simulink model "ImpedanceControl"  (R2020b)
settings: Solver=VariableStepAuto  StartTime=0.0  StopTime=10.0  RelTol=1e-3
libraries: simulink x1
settings Model: Creator=vac  LastModifiedBy=vac

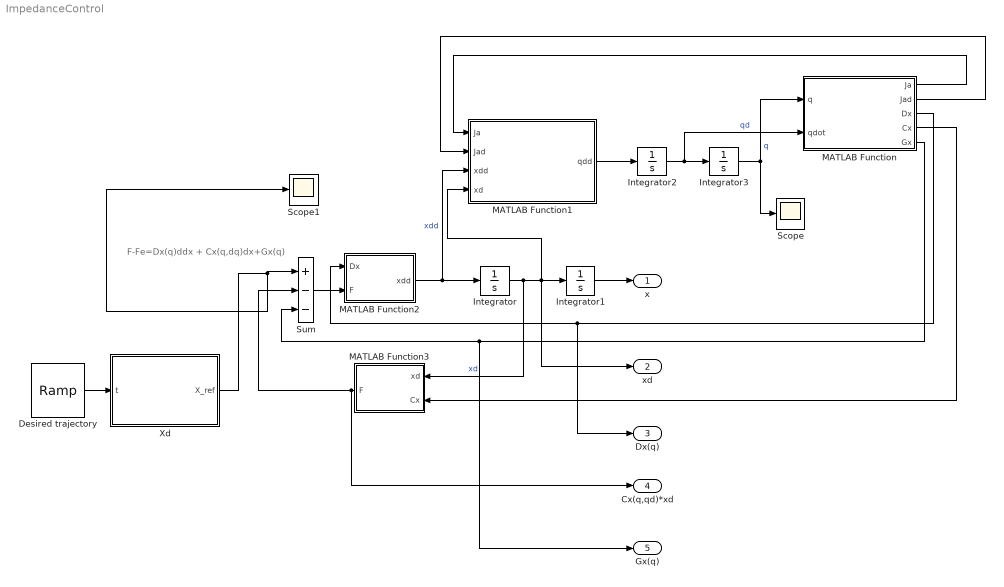
== system ImpedanceControl ==
  note: F-Fe=Dx(q)ddx + Cx(q,dq)dx+Gx(q)
  Desired trajectory : simulink/Sources/Ramp  slope=0.1  start=0  InitialOutput=0
  Integrator : Integrator  InitialCondition=[0;0;0]
  Integrator1 : Integrator  InitialCondition=[0 0 0]'
  Integrator2 : Integrator  InitialCondition=[0 0 0]'
  Integrator3 : Integrator  InitialCondition=[0.1 0.1 0.1]'
  MATLAB Function : MATLAB Function  TreatAsAtomicUnit=on
  MATLAB Function1 : MATLAB Function  TreatAsAtomicUnit=on
  MATLAB Function2 : MATLAB Function  TreatAsAtomicUnit=on
  MATLAB Function3 : MATLAB Function  TreatAsAtomicUnit=on
  Scope : Scope
  Scope1 : Scope
  Sum : Sum  Inputs=+--
  Xd : MATLAB Function  TreatAsAtomicUnit=on
  x : Outport
  xd : Outport  Port=2
  Dx(q) : Outport  Port=3
  Cx(q,qd)*xd : Outport  Port=4
  Gx(q) : Outport  Port=5
  wires:
  MATLAB Function2/1(xdd) -> MATLAB Function1/3(xdd), Integrator/1  "xdd"
  Integrator/1 -> MATLAB Function3/1(xd), xd/1, MATLAB Function1/4(xd), Integrator1/1  "xd"
  Integrator1/1 -> x/1
  MATLAB Function1/1(qdd) -> Integrator2/1
  Integrator2/1 -> MATLAB Function/2(qdot), Integrator3/1  "qd"
  Integrator3/1 -> MATLAB Function/1(q), Scope/1  "q"
  MATLAB Function/1(Ja) -> MATLAB Function1/1(Ja)
  MATLAB Function/2(Jad) -> MATLAB Function1/2(Jad)
  MATLAB Function/3(Dx) -> Dx(q)/1, MATLAB Function2/1(Dx)
  MATLAB Function/4(Cx) -> MATLAB Function3/2(Cx)
  Xd/1(X_ref) -> Sum/1, Scope1/1
  MATLAB Function/5(Gx) -> Gx(q)/1, Sum/3
  Sum/1 -> MATLAB Function2/2(F)
  MATLAB Function3/1(F) -> Cx(q,qd)*xd/1, Sum/2
  Desired trajectory/1 -> Xd/1(t)

== matlab function ImpedanceControl/MATLAB Function1 ==
  data: Ja input; Jad input; xdd input; qdd output; xd input
function qdd = qdoubledot(Ja,Jad,xdd,xd)
qdd = Ja\xdd - inv(Ja)*Jad*inv(Ja)*xd;

== matlab function ImpedanceControl/MATLAB Function ==
  data: Ja output; Jad output; q input; Dx output; Cx output; Gx output; qdot input
function [Ja,Jad,Dx,Cx,Gx] = jacobian_cal(q, qdot)
    q1 = q(1);
    q2 = q(2);
    q3 = q(3);
    qd1 = qdot(1);
    qd2 = qdot(2);
    qd3 = qdot(3);

    % Parameters
    m1 = 3.92; %kg
    m2 = 2.16;
    m3 = 1;

    % link length

    l1 = 0.4; % meter
    l2 = 0.3;
    l3 = 0.2;
    
    g = 9.8;
    % inertia tensor
    Ic1xx = 0.0587; % kg*meter^2
    Ic1yy = 0.0128;
    Ic1zz = 0.0587;

    Ic2xx = 0.0052;
    Ic2yy = 0.0188;
    Ic2zz = 0.0188;

    Ic3xx = 0.0016;
    Ic3yy = 0.0042;
    Ic3zz = 0.0042;


    % Dq
    q23 = q2+q3;
    d11 = Ic1yy + m2*l2^2*cos(q2)^2/4 + Ic2xx*sin(q2)^2 + ...
          Ic2yy*cos(q2)^2 + m3*l2^2*cos(q2)^2 + m3*l3^2*cos(q23)^2/4 + ...
          m3*l2*l3*cos(q2)*cos(q23)+ Ic3xx*sin(q23)^2 + Ic3yy*cos(q23)^2;

    d22 = m2*l2^2/4 + Ic2zz + m3*l2^2 +...
          m3*l3^2/4 + m3*l2*l3*cos(q3) + Ic3zz;
    d23 = m3*l3^2/4 + m3*l2*l3*cos(q3)/2 + Ic3zz;
    d33 = m3*l3^2/4 + Ic3zz;
    Dq  = [d11,   0,   0;
           0,   d22, d23;
           0,   d23, d33];

    % Cq
    h1 = sin(q2+q2)*(-m2*l2^2/4 + Ic2xx -Ic2yy - m3*l2^2) + ...
         sin(q2*2+q3*2)*(-m3*l3^2/4 + Ic3xx - Ic3yy) - sin(q2+q2+q3)*m3*l2*l3;
    h2 = sin(q2*2+q3*2)*(-m3*l3^2/4 + Ic3xx - Ic3yy) - cos(q2)*sin(q23)*m3*l2*l3;
    h3 = -sin(q3)*m3*l2*l3;
    Cq = 0.5*[h1*qd2 + h2*qd3,  h1*qd1, h2*qd1;
                     - h1*qd1,  h3*qd3, h3*qd2 + h3*qd3;
                     - h2*qd1, -h3*qd2, 0];
    % Gq
    Gq = [ 0;
          -m2*g*l2*cos(q2)/2 - m3*g*l2*cos(q2) - m3*g*l3*cos(q23)/2;
          -m3*g*l3*cos(q23)/2];

    % Analytical Jacobian
    j11 = -l2*sin(q1)*cos(q2)-l3*sin(q1)*cos(q23);
    j12 = -l2*cos(q1)*sin(q2)-l3*cos(q1)*sin(q2+q3);
    j13 = -l3*cos(q1)*sin(q23);
    j21 = l2*cos(q1)*cos(q2)+l3*cos(q1)*cos(q23);
    j22 = -l2*sin(q1)*sin(q2)-l3*sin(q1)*cos(q23);
    j23 = -l3*sin(q1)*sin(q23);
    j31 = 0;
    j32 = -l2*cos(q2)-l3*cos(q23);
    j33 = -3*cos(q23);
    Ja = [j11, j12, j13;
          j21, j22, j23;
          j31, j32, j33];

    % Analytical jacobian dot
    jd11 = -l2*cos(q1)*cos(q2)*qd1   + l2*sin(q1)*sin(q2)*qd2 ...
           - l3*cos(q1)*cos(q23)*qd1 + l3*sin(q1)*sin(q23)*(qd2+qd3);
    jd12 = l2*sin(q1)*sin(q2)*qd1    - l2*cos(q1)*cos(q2)*qd2...
           + l3*sin(q1)*sin(q23)*qd1 - l3*cos(q1)*cos(q23)*(qd2+qd3);
    jd13 = l3*sin(q1)*sin(q23)*qd1   - l3*cos(q1)*cos(q23)*(qd2+qd3);
    jd21 = - l2*sin(q1)*cos(q2)*qd1  - l2*cos(q1)*sin(q2)*qd2...
           - l3*sin(q1)*cos(q23)*qd1 - l3*cos(q1)*sin(q23)*(qd2+qd3);
    jd22 = -l2*cos(q1)*sin(q2)*qd1   - l2*sin(q1)*cos(q2)*qd2...
           - l3*cos(q1)*sin(q23)*qd1 - l3*sin(q1)*cos(q23)*(qd2+qd3);
    jd23 = -l3*cos(q1)*sin(q23)*qd1  - l3*sin(q1)*cos(q23)*(qd2+qd3);
    jd31 = 0;
    jd32 = l2*sin(q2)*qd2 + l3*sin(q23)*(qd2+qd3);
    jd33 = l3*sin(q23)*(qd2+qd3);
    Jad  = [ jd11, jd12, jd13;
             jd21, jd22, jd23;
             jd31, jd32, jd33];
    % inverse transpose     
    Jait = inv(Ja)';
    Dx = Jait*Dq/Ja;
    Cx = Jait*(Cq - Dq/Ja*Jad)/Ja;
    Gx = Jait*Gq;

== matlab function ImpedanceControl/MATLAB Function2 ==
  data: Dx input; xdd output; F input
function xdd = fcn(Dx,F)
xdd = Dx\F;

== matlab function ImpedanceControl/MATLAB Function3 ==
  data: xd input; F output; Cx input
function F = fcn(xd,Cx)

F=Cx*xd;

== matlab function ImpedanceControl/Xd ==
  data: t input; X_ref output
function X_ref  = fcn(t)

x_ref = 0.1 + 0.05 * t;% + 0.1*sin(7*t);
y_ref = 0.3 - 0.05*t;
z_ref = 0.5 + 0.05*t;

X_ref = [x_ref,y_ref,z_ref]';
